simulink model "UKF_EKF_XY"  (R2020b)
settings: Solver=ode45  StartTime=0.0  StopTime=180  FixedStep=1e-7  RelTol=1e-4  AbsTol=1e-4  EnableMultiTasking=on
libraries: simulink x3
settings Model: Creator=André  LastModifiedBy=Andre
settings SolverCC: AutoScaleAbsTol=off  ConsecutiveZCsStepRelTol=100*128*eps  ShapePreserveControl=EnableAll  ZeroCrossControl=EnableAll  AutoInsertRateTranBlk=on
settings DataIOCC: LimitDataPoints=on  SaveFormat=Array  SignalLoggingSaveFormat=ModelDataLogs  ReturnWorkspaceOutputs=off
settings OptimizationCC: ExpressionDepthLimit=2147483647  LifeSpan=inf
settings DebuggingCC: UnderspecifiedInitializationDetection=Classic  MergeDetectMultiDrivingBlocksExec=none  SolverPrmCheckMsg=warning  FcnCallInpInsideContextMsg=warning  StateNameClashWarn=warning  SFUnexpectedBacktrackingDiag=warning  SFNoUnconditionalDefaultTransitionDiag=warning  SFExecutionAtInitializationDiag=none  ArithmeticOperatorsInVariantConditions=warning
settings HardwareCC: ProdBitPerPointer=32  ProdBitPerSizeT=32  ProdBitPerPtrDiffT=32  ProdLargestAtomicFloat=None  ProdIntDivRoundTo=Undefined  ProdEndianess=Unspecified  ProdWordSize=32  ProdHWDeviceType=32-bit Generic
settings ModelReferenceCC: PropagateSignalLabelsOutOfModel=off
settings SFSimCC: SimUseLocalCustomCode=off  SimParseCustomCode=off  CustomCodeUndefinedFunction=UseInterfaceOnly
settings RTWCC: RTWUseLocalCustomCode=off
settings CodeAppCC: StateflowObjectComments=on
settings GRTTargetCC: TargetLangStandard=C89/C90 (ANSI)  CombineOutputUpdateFcns=off  GRTInterface=on
settings ConfigComp: CovMetricSettings=dw  CovSaveCumulativeToWorkspaceVar=on  CovSaveSingleToWorkspaceVar=on  CovExternalEMLEnable=off

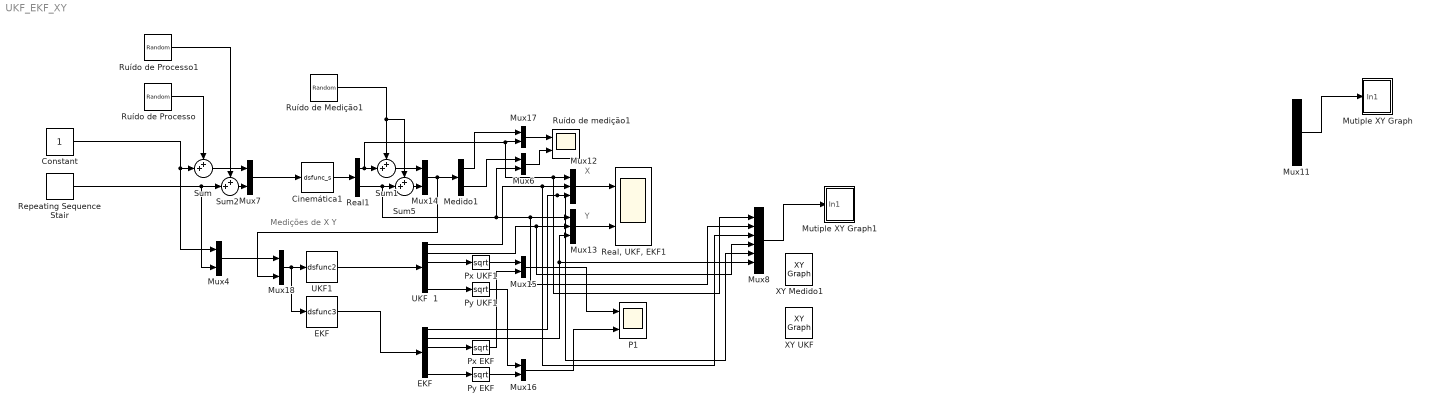
== system UKF_EKF_XY ==
  note: X
  note: Medições de X Y
  note: Y
  Cinemática1 : S-Function  FunctionName=dsfunc_s  Parameters=[0 0]  SFunctionDeploymentMode=off  EnableBusSupport=off
  Constant : Constant
  EKF : S-Function  FunctionName=dsfunc3  Parameters=[-10 -10 100 0 0 100]  SFunctionDeploymentMode=off  EnableBusSupport=off
  "EKF " : Demux  Outputs=6
  Medido1 : Demux  Outputs=2
  Mutiple XY Graph : Subsystem  mask(Mutiple XY Graph){number_of_trajectories=3, axis_limits=[-200 200 -200 200], sample_time=0.1}
      mask prompts: number_of_trajectories "Number of Trajectories"; axis_limits "Axis Limits"; sample_time "Sample Time"
      mask Display: plot([.05 .95 .95 .05 .05],[.45 .45 .95 .95 .45], 0.5+cos(0:0.1:2*pi)*0.3,0.7+sin(0:0.1:2*pi)*0.2)
  Mutiple XY Graph1 : Subsystem  mask(Mutiple XY Graph){number_of_trajectories=3, axis_limits=[-200 200 -200 200], sample_time=0.1}
      mask prompts: number_of_trajectories "Number of Trajectories"; axis_limits "Axis Limits"; sample_time "Sample Time"
      mask Display: plot([.05 .95 .95 .05 .05],[.45 .45 .95 .95 .45], 0.5+cos(0:0.1:2*pi)*0.3,0.7+sin(0:0.1:2*pi)*0.2)
  Mux11 : Mux  Inputs=6
  Mux12 : Mux  Inputs=3
  Mux13 : Mux  Inputs=3
  Mux{4,6..7,14..18} (8 alike) : Mux  Inputs=2
  Mux8 : Mux  Inputs=6
  P1 : Scope  NumInputPorts=2
  Px EKF : Sqrt  SaturateOnIntegerOverflow=on
  Px UKF1 : Sqrt  SaturateOnIntegerOverflow=on
  Py EKF : Sqrt  SaturateOnIntegerOverflow=on
  Py UKF1 : Sqrt  SaturateOnIntegerOverflow=on
  "Real, UKF, EKF1" : Scope  NumInputPorts=2
  Real1 : Demux  Outputs=2
  Repeating Sequence Stair : simulink/Sources/Repeating Sequence Stair  OutValues="[0 pi/4 2*pi/4 3*pi/4 pi 5*pi/4  6*pi/4 7*pi/4  ].'"  tsamp=20  OutMin=[]  OutMax=[]  OutDataTypeStr=double  OutputDataTypeScalingMode=double  OutDataType=fixdt(0,8)  ConRadixGroup=Best Precision: Vector-wise  OutScaling=2^-12
  Ruído de Medição1 : RandomNumber  SampleTime=0.01
  Ruído de Processo : RandomNumber  SampleTime=0.01
  Ruído de Processo1 : RandomNumber  Variance=0.6  SampleTime=0.01
  Ruído de medição1 : Scope  NumInputPorts=2
  Sum{,1..2,5} (4 alike) : Sum  Inputs=++|
  UKF  1 : Demux  Outputs=6
  UKF1 : S-Function  FunctionName=dsfunc2  Parameters=[-10 -10 100 0 0 100]  SFunctionDeploymentMode=off  EnableBusSupport=off
  XY Medido1 : simulink/Sinks/XY Graph  xmin=-200  xmax=200  ymin=-200  ymax=200  st=-1
  XY UKF : simulink/Sinks/XY Graph  xmin=-200  xmax=200  ymin=-200  ymax=200  st=-1
  wires:
  Ruído de Processo/1 -> Sum/1
  Sum2/1 -> Mux7/2
  Constant/1 -> Mux4/1, Sum/2
  Sum/1 -> Mux7/1
  Mux11/1 -> Mutiple XY Graph/1(In1)
  Repeating Sequence Stair/1 -> Mux4/2, Sum2/2
  Ruído de Processo1/1 -> Sum2/1
  "EKF "/2 -> Mux13/3, Mux8/6
  Mux15/1 -> P1/1
  Mux6/1 -> Ruído de medição1/2
  UKF  1/6 -> Py UKF1/1
  Mux17/1 -> Ruído de medição1/1
  Mux16/1 -> P1/2
  Mux8/1 -> Mutiple XY Graph1/1(In1)
  Real1/1 -> Mux8/1, Mux12/1, Mux17/2, Sum1/2
  Medido1/2 -> Mux6/1
  Mux14/1 -> Mux18/2, Medido1/1
  "EKF "/1 -> Mux8/5, Mux12/3
  Py EKF/1 -> Mux16/2
  Sum5/1 -> Mux14/2
  Medido1/1 -> Mux17/1
  Px EKF/1 -> Mux15/2
  EKF/1 -> "EKF "/1
  Px UKF1/1 -> Mux15/1
  "EKF "/3 -> Px EKF/1
  UKF  1/1 -> Mux8/3, Mux12/2
  UKF1/1 -> UKF  1/1
  Mux12/1 -> "Real, UKF, EKF1"/1
  Real1/2 -> Mux8/2, Mux13/1, Mux6/2, Sum5/2
  Mux13/1 -> "Real, UKF, EKF1"/2
  UKF  1/3 -> Px UKF1/1
  Cinemática1/1 -> Real1/1
  Sum1/1 -> Mux14/1
  "EKF "/6 -> Py EKF/1
  Mux7/1 -> Cinemática1/1
  Py UKF1/1 -> Mux16/1
  Ruído de Medição1/1 -> Sum1/1, Sum5/1
  UKF  1/2 -> Mux8/4, Mux13/2
  Mux18/1 -> EKF/1, UKF1/1
  Mux4/1 -> Mux18/1

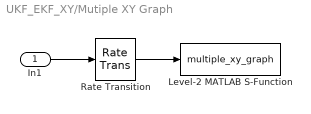
== system UKF_EKF_XY/Mutiple XY Graph ==
  In1 : Inport
  Level-2 MATLAB S-Function : M-S-Function  FunctionName=multiple_xy_graph  Parameters=number_of_trajectories,axis_limits
  Rate Transition : RateTransition  OutPortSampleTime=sample_time
  wires:
  In1/1 -> Rate Transition/1
  Rate Transition/1 -> Level-2 MATLAB S-Function/1

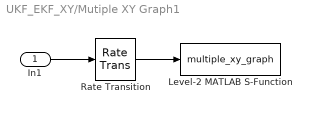
== system UKF_EKF_XY/Mutiple XY Graph1 ==
  In1 : Inport
  Level-2 MATLAB S-Function : M-S-Function  FunctionName=multiple_xy_graph  Parameters=number_of_trajectories,axis_limits
  Rate Transition : RateTransition  OutPortSampleTime=sample_time
  wires:
  In1/1 -> Rate Transition/1
  Rate Transition/1 -> Level-2 MATLAB S-Function/1
